simulink model "udp_conn"  (R2018b)
settings: Solver=FixedStepDiscrete  StartTime=0.0  StopTime=2*3600  RelTol=1e-3  EnableMultiTasking=on
model workspace (MATLAB code in the model file):
  | %load('../subsystems/mpc_30min_P1day.mat')
  | % load('labsys_mpc_v0.3_20sec.mat')
  | % load('labsys_mpc_v0.5.mat')
  | % load('labsys_mpc_v0.6.mat')
  | % load('labsys_mpc_v0.7.mat')
  | % load('labsys_mpc_v0.8.mat')
  | % load('labsys_mpc_v0.9.mat')
  | load('mpc_param_var05_duweight.mat')
undefined symbols (not defined in the file or in its folder): refA, refB, sldrtexcb_modeswitch, Standard_Devices, Ts, UDP_Protocol
libraries: mpclib x4, simulink x2, sldrtlib x2
Description:
  | Packet Input/Output
  | 
  | The example model "sldrtex_packetio" shows how to transfer data through UDP
  | communication protocol using binary encoding. The model sends data
  | within one computer, from one UDP port to another. You can modify the
  | model to communicate between two computers by splitting this model
  | into its send and receive parts and running the models on two computers.
  | The yellow blocks are used to send the data, the blue blocks
  | are used to receive the data. Then, please enter the IP addresses of the two
  | computers into the appropriate fields in the Board Setup dialog.
  | 
  | How to run this model in Normal Mode:
  | 
  | 1) Double-click the orange button to switch to Normal Mode if needed.
  | 2) Start the real-time execution using Simulation->Run.
  | 
  | How to run this model in External Mode:
  | 
  | 1) Double-click the orange button to switch to External Mode if needed.
  | 2) Start the real-time execution using Simulation->Run. The model will automatically
  |    build, connect to Simulink in External Mode and start.
settings Model: SimulationMode=external  ExtModeTrigDuration=1001  ExtModeArchiveMode=auto  ExtModeArchiveFileName=labsys_data  ExtModeArchiveDirName=C:\Users\gylaszlo.SCH\Documents\szakdoga\thesis\model\real_sys\data  ExtModeAddSuffixToVar=on  ExtModeWriteAllDataToWs=on  Creator=The MathWorks, Inc.  LastModifiedBy=gylaszlo
settings DataIOCC: LimitDataPoints=on  SaveFormat=Array
settings OptimizationCC: ExpressionDepthLimit=2147483647  InitFltsAndDblsToZero=on  EfficientMapNaN2IntZero=off  LifeSpan=inf
settings DebuggingCC: UnderspecifiedInitializationDetection=Classic  MergeDetectMultiDrivingBlocksExec=none  SolverPrmCheckMsg=warning  FcnCallInpInsideContextMsg=warning  AllowSymbolicDim=off  StateNameClashWarn=warning  SFUnexpectedBacktrackingDiag=warning  SFNoUnconditionalDefaultTransitionDiag=warning  SFExecutionAtInitializationDiag=none
settings HardwareCC: TargetBitPerLong=64  TargetBitPerPointer=64  TargetBitPerSizeT=64  TargetBitPerPtrDiffT=64  TargetIntDivRoundTo=Zero  TargetEndianess=LittleEndian  TargetWordSize=64  TargetHWDeviceType=Intel->x86-64
settings ModelReferenceCC: PropagateSignalLabelsOutOfModel=off
settings SFSimCC: SimUseLocalCustomCode=off
settings RTWCC: SystemTargetFile=sldrt.tlc  TemplateMakefile=sldrt.tmf  Description=Simulink Desktop Real-Time  RTWUseLocalCustomCode=off  RTWCompilerOptimization=on
settings CodeAppCC: MaxIdLength=95  StateflowObjectComments=on
settings SimulinkDesktopRealTimeCC: TargetPreCompLibLocation=C:\Program Files\MATLAB\R2018b\toolbox\sldrt\lib\win64  TargetLangStandard=C89/C90 (ANSI)  GeneratePreprocessorConditionals=Disable all  SupportVariableSizeSignals=off  PreserveStateflowLocalDataDimensions=off
settings ConfigComp: CovMetricSettings=dw  CovHtmlReporting=on  CovSaveCumulativeToWorkspaceVar=on  CovSaveSingleToWorkspaceVar=on  CovShowResultsExplorer=off  CovExternalEMLEnable=off  CovSFcnEnable=off

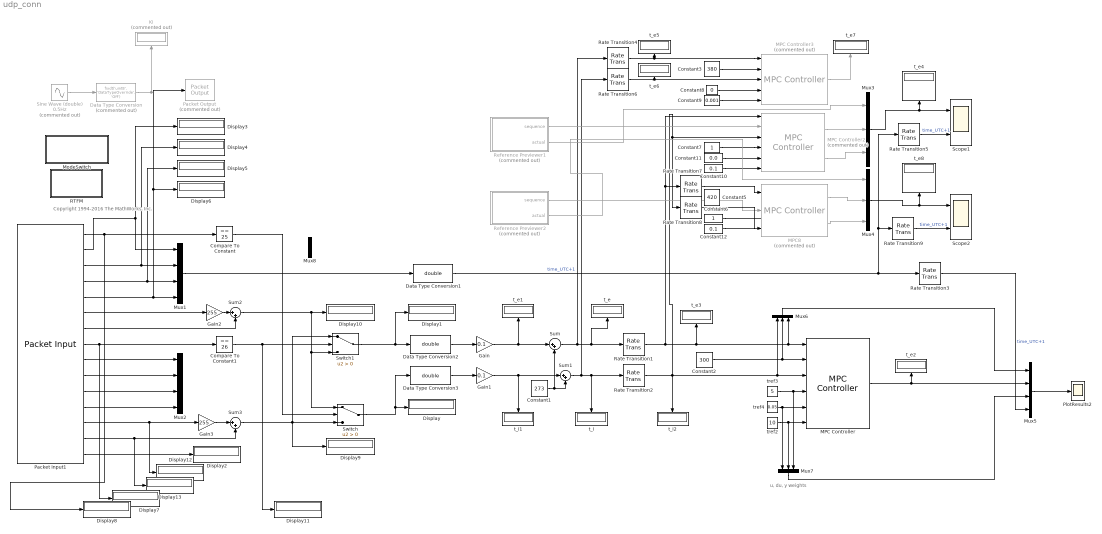
== system udp_conn ==
  note: u, du, y weights
  note: Copyright 1994-2016 The MathWorks, Inc.
  Compare To Constant : simulink/Logic and Bit Operations/Compare To Constant  relop===  const=25  OutDataTypeStr=uint8
  Compare To Constant1 : simulink/Logic and Bit Operations/Compare To Constant  relop===  const=26  OutDataTypeStr=uint8
  Constant1 : Constant  Value=273
  Constant10 : Constant  Value=0.1
  Constant11 : Constant  Value=0.0
  Constant12 : Constant  Value=0.1
  Constant2 : Constant  Value=300
  Constant3 : Constant  Value=380
  Constant5 : Constant  Value=420
  Constant6 : Constant
  Constant7 : Constant
  Constant8 : Constant  Value=0
  Constant9 : Constant  Value=0.001
  Data Type Conversion : DataTypeConversion  Commented=on  OutDataTypeStr=fixdt('uint8', 'DataTypeOverride', 'Off')  RndMeth=Nearest  SaturateOnIntegerOverflow=on
  Data Type Conversion1 : DataTypeConversion  OutDataTypeStr=double  RndMeth=Nearest  SaturateOnIntegerOverflow=on
  Data Type Conversion2 : DataTypeConversion  OutDataTypeStr=double  RndMeth=Nearest  SaturateOnIntegerOverflow=on
  Data Type Conversion3 : DataTypeConversion  OutDataTypeStr=double  RndMeth=Nearest  SaturateOnIntegerOverflow=on
  Display{,1..13} (14 alike) : Display
      Display settings: Format=hex (Stored Integer)
      Display1 settings: Format=hex (Stored Integer)
      Display10 settings: Format=hex (Stored Integer)
      Display11 settings: Format=hex (Stored Integer)
      Display12 settings: Format=decimal (Stored Integer)
      Display13 settings: Format=decimal (Stored Integer)
      Display2 settings: Format=hex (Stored Integer)
      Display3 settings: Format=decimal (Stored Integer)
      Display4 settings: Format=decimal (Stored Integer)
      Display5 settings: Format=decimal (Stored Integer)
      Display6 settings: Format=decimal (Stored Integer)
      Display7 settings: Format=decimal (Stored Integer)
      Display8 settings: Format=decimal (Stored Integer)
      Display9 settings: Format=hex (Stored Integer)
  Gain : Gain  Gain=0.1
  Gain1 : Gain  Gain=0.1
  Gain2 : Gain  Gain=255
  Gain3 : Gain  Gain=255
  Ki : Display  Commented=on
  MPC Controller : mpclib/MPC Controller  SCDEnableBlockLinearizationSpecification=on  mpcobj=mpc_labsys05_du10  x0=mpcstate05  is_multiple=0  enable_value=0  return_u0=off  updateMPCinCallerWorkspace=on  md_inport=on  mv_inport=off  return_cost=off  return_mvseq=off  return_qpstatus=off  return_xseq=off  return_state=off  return_ovseq=off  state_inport=off  umin_inport=off  umax_inport=off  ymin_inport=off  ymax_inport=off  cc_inport=off  ywt_inport=on  uwt_inport=on  duwt_inport=on  rhoeps_inport=off  uref_inport=off  n_ts=30  n_p=100  n_mv=1  n_md=1  n_ud=0  n_mo=1  n_uo=0  BlockDataType=double  SampleTimeInherited=off  switch_inport=off
  MPC Controller2 : mpclib/MPC Controller  Commented=on  SCDEnableBlockLinearizationSpecification=on  mpcobj=mpc_labsys09  is_multiple=0  enable_value=0  return_u0=off  updateMPCinCallerWorkspace=on  md_inport=on  mv_inport=off  return_cost=on  return_mvseq=off  return_qpstatus=off  return_xseq=off  return_state=off  return_ovseq=off  state_inport=off  umin_inport=off  umax_inport=off  ymin_inport=off  ymax_inport=off  cc_inport=off  ywt_inport=on  uwt_inport=on  duwt_inport=on  rhoeps_inport=off  uref_inport=off  n_ts=20  n_p=50  n_mv=1  n_md=1  n_ud=0  n_mo=1  n_uo=0  BlockDataType=double  SampleTimeInherited=off  switch_inport=off
  MPC Controller3 : mpclib/MPC Controller  Commented=on  SCDEnableBlockLinearizationSpecification=on  mpcobj=mpc_labsys05  is_multiple=0  enable_value=0  return_u0=off  updateMPCinCallerWorkspace=on  md_inport=on  mv_inport=off  return_cost=off  return_mvseq=off  return_qpstatus=off  return_xseq=off  return_state=off  return_ovseq=off  state_inport=off  umin_inport=off  umax_inport=off  ymin_inport=off  ymax_inport=off  cc_inport=off  ywt_inport=on  uwt_inport=on  duwt_inport=off  rhoeps_inport=off  uref_inport=off  n_ts=30  n_p=100  n_mv=1  n_md=1  n_ud=0  n_mo=1  n_uo=0  BlockDataType=double  SampleTimeInherited=off  switch_inport=off
  MPC8 : mpclib/MPC Controller  Commented=on  SCDEnableBlockLinearizationSpecification=on  mpcobj=mpc_labsys11  is_multiple=0  enable_value=0  return_u0=off  updateMPCinCallerWorkspace=on  md_inport=on  mv_inport=off  return_cost=on  return_mvseq=off  return_qpstatus=off  return_xseq=off  return_state=off  return_ovseq=off  state_inport=off  umin_inport=off  umax_inport=off  ymin_inport=off  ymax_inport=off  cc_inport=off  ywt_inport=off  uwt_inport=off  duwt_inport=off  rhoeps_inport=off  uref_inport=off  n_ts=300  n_p=10  n_mv=1  n_md=1  n_ud=0  n_mo=1  n_uo=0  BlockDataType=double  SampleTimeInherited=off  switch_inport=off
  ModeSwitch : Subsystem  InitFcn=sldrtexcb_modeswitch('CheckKernel');  mask(Simulink Desktop Real-Time Example Mode Switch){}
      settings: OpenFcn=sldrtexcb_modeswitch(gcbh);
      mask Display: disp('Switch To\nNormal Mode');
  Mux1 : Mux
  Mux2 : Mux
  Mux{3..4,6..7} (4 alike) : Mux  Inputs=3
  Mux5 : Mux
  Mux8 : Mux  Inputs=2
  Packet Input1 : sldrtlib/Packet Input  SampleTime=1  MaxMissedTicks=10  ShowMissedTicks=on  YieldWhenWaiting=on  DrvName=Standard_Devices/UDP_Protocol  DrvAddress=9089  DrvOptions=[0 9090 49 57 50 46 49 54 56 46 48 46 49 48 56 0 0 0 0 0 0 0 0 0 0 0 0 0 0 0 0 0 0 0 0 0 0 0 0 0 0 0 0 0 0 0 0 0 0 0 0 0 0 0 0 0 0 0 0 0 0 0 0 0 0 0 0 0 0 0 0 0 0 0 0 0 0 0 0 0 0 0 0 0 0 0 0 0 0 0 0 0 0 0 0 0 0 0 0 0 0 0 0 0 0 0 0 0 0 0 0 0 0 0 0 0 0 0 0 0 0 0 0 0 0 0 0 0 0 0 0 0 0 0 0 0 0 0 0 0 0 0 0 0 0 0 0 0 0 0 0 0 0 0 0 0 0 0 0 0 0 0 0 0 0 0 0 0 0 0 0 0 0 0 0 0 0 0 0 0 0 0 0 0 0 0 0 0 0 0 0 0 0 0 0 0 0 0 0 0 0 0 0 0 0 0 0 0 0 0 0 0 0 0 0 0 0 0 0 0 0 0 0 0 0 0 0 0 0 0 0 0 0 0 0 0 0 0 0 0 0 0 0 0 0 0 0 0 0 0 0 0 0 0 0 0]  PacketSize=14  DataTypes={'uint8','uint8','uint8','uint8','uint8','uint8','uint8','uint8','uint8','uint8','uint8','uint8','uint8','uint8'}  ShowReady=off  ShowError=off  PacketID=1  ByteOrder=1  ShowTimestamp=off
      settings: AttributesFormatString=UDP Protocol [9089]  SourceProductName=Simulink Desktop Real-Time
  Packet Output : sldrtlib/Packet Output  Commented=on  SampleTime=1  MaxMissedTicks=50  ShowMissedTicks=off  YieldWhenWaiting=off  DrvName=Standard_Devices/UDP_Protocol  DrvAddress=9089  DrvOptions=[0 9090 49 54 56 46 49 57 50 46 48 46 49 48 56 0 0 0 0 0 0 0 0 0 0 0 0 0 0 0 0 0 0 0 0 0 0 0 0 0 0 0 0 0 0 0 0 0 0 0 0 0 0 0 0 0 0 0 0 0 0 0 0 0 0 0 0 0 0 0 0 0 0 0 0 0 0 0 0 0 0 0 0 0 0 0 0 0 0 0 0 0 0 0 0 0 0 0 0 0 0 0 0 0 0 0 0 0 0 0 0 0 0 0 0 0 0 0 0 0 0 0 0 0 0 0 0 0 0 0 0 0 0 0 0 0 0 0 0 0 0 0 0 0 0 0 0 0 0 0 0 0 0 0 0 0 0 0 0 0 0 0 0 0 0 0 0 0 0 0 0 0 0 0 0 0 0 0 0 0 0 0 0 0 0 0 0 0 0 0 0 0 0 0 0 0 0 0 0 0 0 0 0 0 0 0 0 0 0 0 0 0 0 0 0 0 0 0 0 0 0 0 0 0 0 0 0 0 0 0 0 0 0 0 0 0 0 0 0 0 0 0 0 0 0 0 0 0 0 0 0 0 0 0 0 0]  PacketSize=1  DataTypes={'uint8'}  ShowReady=off  ShowError=off  PacketID=1  ByteOrder=1  InitialValue=0  FinalValue=[]
      settings: AttributesFormatString=UDP Protocol [9089]  SourceProductName=Simulink Desktop Real-Time
  PlotResults2 : Scope
  "RTFM " : Subsystem  mask(Simulink Desktop Real-Time Example Info){}
      settings: OpenFcn=web([docroot '/sldrt/examples/packet-input-output.html']);
      mask Display: disp('Info')
  Rate Transition1 : RateTransition  Integrity=off  Deterministic=off  OutPortSampleTime=30
  Rate Transition2 : RateTransition  Integrity=off  OutPortSampleTime=30
  Rate Transition3 : RateTransition  Integrity=off  OutPortSampleTime=30
  Rate Transition4 : RateTransition  Integrity=off  Deterministic=off  OutPortSampleTime=30
  Rate Transition5 : RateTransition  Integrity=off  OutPortSampleTime=20
  Rate Transition6 : RateTransition  Integrity=off  OutPortSampleTime=30
  Rate Transition7 : RateTransition  Integrity=off  Deterministic=off  OutPortSampleTime=300
  Rate Transition8 : RateTransition  Integrity=off  Deterministic=off  OutPortSampleTime=300
  Rate Transition9 : RateTransition  Integrity=off  OutPortSampleTime=300
  Reference Previewer1 : Subsystem  Commented=on  mask{signal=refA, ts=20, steps=50}
      mask prompts: signal "Signal name"; ts "Sampling time"; steps "Number of previewing steps"
      mask init:
      | ts = evalin('base',get_param(gcbh,'ts'));
      | signal = evalin('base',get_param(gcbh,'signal'));
      | steps = evalin('base',get_param(gcbh,'steps'));
      | data = mpc_previewer_maskinit(signal,ts);
      mask Display:
      | fprintf('Future\nsample\nextractor');
      | port_label('output', 1, 'seq')
      | port_label('output', 2, '@t')
  Reference Previewer2 : Subsystem  Commented=on  mask{signal=refB, ts=Ts, steps=10}
      mask prompts: signal "Signal name"; ts "Sampling time"; steps "Number of previewing steps"
      mask init:
      | ts = evalin('base',get_param(gcbh,'ts'));
      | signal = evalin('base',get_param(gcbh,'signal'));
      | steps = evalin('base',get_param(gcbh,'steps'));
      | data = mpc_previewer_maskinit(signal,ts);
      mask Display:
      | fprintf('Future\nsample\nextractor');
      | port_label('output', 1, 'seq')
      | port_label('output', 2, '@t')
  Scope1 : Scope  NumInputPorts=2
  Scope2 : Scope  NumInputPorts=2
  Sine Wave (double) 0.5Hz : Sin  Commented=on  Amplitude=50  Bias=50  Frequency=0.62*0.5  SampleTime=1
  Sum{,1..3} (4 alike) : Sum  Inputs=|++
  Switch : Switch  Criteria=u2 > Threshold
  Switch1 : Switch  Criteria=u2 > Threshold
  t_e{,1..8} (9 alike) : Display
  t_i : Display
  t_i1 : Display
  t_i2 : Display
  tref2 : Constant  Value=10  SampleTime=30
  tref3 : Constant  Value=5  SampleTime=30
  tref4 : Constant  Value=0.05  SampleTime=30
  wires:
  Data Type Conversion/1 -> Ki/1
  Data Type Conversion2/1 -> Gain/1
  Sine Wave (double) 0.5Hz/1 -> Data Type Conversion/1
  MPC Controller/1 -> t_e2/1, Mux5/2
  Gain/1 -> Sum/1, t_e1/1
  Data Type Conversion3/1 -> Gain1/1
  Gain1/1 -> Sum1/1, t_i1/1
  Constant1/1 -> Sum1/2, Sum/2
  Switch/1 -> Data Type Conversion3/1, Display/1
  Constant2/1 -> MPC Controller/2, Mux6/2
  Switch1/1 -> Data Type Conversion2/1, Display1/1
  Gain2/1 -> Sum2/1
  Packet Input1/6 -> Gain2/1
  Packet Input1/7 -> Sum2/2
  Packet Input1/13 -> Gain3/1, Display12/1
  Gain3/1 -> Sum3/1
  Packet Input1/14 -> Display13/1, Sum3/2
  Packet Input1/15 -> Display2/1
  Packet Input1/2 -> Mux1/1, Display3/1
  Packet Input1/3 -> Mux1/2, Display4/1
  Packet Input1/4 -> Mux1/3, Display5/1
  Mux1/1 -> Data Type Conversion1/1
  Rate Transition3/1 -> Mux5/4  "time_UTC+1"
  Packet Input1/5 -> Packet Output/1, Display6/1, Mux1/4
  Packet Input1/9 -> Mux2/1
  Packet Input1/11 -> Mux2/3
  Packet Input1/10 -> Mux2/2
  Packet Input1/12 -> Mux2/4
  Compare To Constant1/1 -> Display11/1, Switch1/2
  Sum3/1 -> Switch1/1, Switch/3, Display9/1
  Packet Input1/1 -> Display8/1, Compare To Constant/1
  Sum2/1 -> Display10/1, Switch1/3, Switch/1
  Packet Input1/8 -> Compare To Constant1/1, Display7/1
  Compare To Constant/1 -> Switch/2
  Sum/1 -> t_e/1, Rate Transition1/1, Rate Transition4/1
  Sum1/1 -> Rate Transition2/1, t_i/1, Rate Transition6/1
  Data Type Conversion1/1 -> Rate Transition3/1, Rate Transition5/1, Rate Transition9/1  "time_UTC+1"
  Rate Transition1/1 -> MPC Controller/1, Mux6/3, t_e3/1, MPC Controller2/1, Rate Transition7/1
  Rate Transition2/1 -> MPC Controller/3, Mux6/1, t_i2/1, Rate Transition8/1, MPC Controller2/3
  MPC Controller2/1 -> Mux3/2
  MPC Controller3/1 -> t_e7/1
  MPC8/1 -> Mux4/2
  Mux3/1 -> t_e4/1, Scope1/1
  Rate Transition4/1 -> MPC Controller3/1, t_e5/1
  Rate Transition5/1 -> Scope1/2  "time_UTC+1"
  Rate Transition6/1 -> MPC Controller3/3, t_e6/1
  Constant3/1 -> MPC Controller3/2
  Constant6/1 -> ?
  Constant7/1 -> MPC Controller2/4
  Constant8/1 -> MPC Controller3/4
  Constant9/1 -> MPC Controller3/5
  Constant10/1 -> MPC Controller2/6
  Constant11/1 -> MPC Controller2/5
  MPC Controller2/2 -> Mux3/3
  Constant12/1 -> ?
  MPC8/2 -> Mux4/3
  Reference Previewer1/2(actual) -> Mux3/1
  Reference Previewer1/1(sequence) -> MPC Controller2/2
  Reference Previewer2/1(sequence) -> MPC8/2
  Reference Previewer2/2(actual) -> Mux4/1
  Rate Transition7/1 -> MPC8/1
  Rate Transition8/1 -> MPC8/3
  Rate Transition9/1 -> Scope2/2  "time_UTC+1"
  Mux4/1 -> Scope2/1, t_e8/1
  tref2/1 -> Mux7/2, MPC Controller/6
  Mux7/1 -> Mux5/3
  Mux6/1 -> Mux5/1
  Mux5/1 -> PlotResults2/1
  tref3/1 -> Mux7/3, MPC Controller/4
  tref4/1 -> Mux7/1, MPC Controller/5

== system udp_conn/ModeSwitch ==

== system udp_conn/RTFM  ==

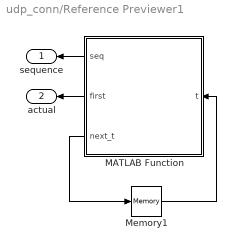
== system udp_conn/Reference Previewer1 ==
  MATLAB Function : MATLAB Function  TreatAsAtomicUnit=on
  Memory1 : Memory  InheritSampleTime=on  LinearizeAsDelay=on
  sequence : Outport
  actual : Outport  Port=2
  wires:
  MATLAB Function/1(seq) -> sequence/1
  Memory1/1 -> MATLAB Function/1(t)
  MATLAB Function/3(next_t) -> Memory1/1
  MATLAB Function/2(first) -> actual/1

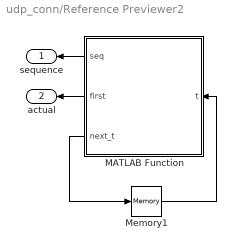
== system udp_conn/Reference Previewer2 ==
  MATLAB Function : MATLAB Function  TreatAsAtomicUnit=on
  Memory1 : Memory  InheritSampleTime=on  LinearizeAsDelay=on
  sequence : Outport
  actual : Outport  Port=2
  wires:
  MATLAB Function/1(seq) -> sequence/1
  Memory1/1 -> MATLAB Function/1(t)
  MATLAB Function/3(next_t) -> Memory1/1
  MATLAB Function/2(first) -> actual/1

== matlab function udp_conn/Reference Previewer2/MATLAB Function ==
  settings: updateMethod=DISCRETE  sampleTime=ts
  data: data parameter double; seq output double; steps parameter double; t input double; first output double; next_t output double
function [seq,first,next_t] = fcn(data,steps,t)
%#codegen
[seq,first,next_t] = mpcblock_preview('ref',data,steps,t);

== matlab function udp_conn/Reference Previewer1/MATLAB Function ==
  settings: updateMethod=DISCRETE  sampleTime=ts
  data: data parameter double; seq output double; steps parameter double; t input double; first output double; next_t output double
function [seq,first,next_t] = fcn(data,steps,t)
%#codegen
[seq,first,next_t] = mpcblock_preview('ref',data,steps,t);
